simulink library "microgridLib"  (R2023a)
settings: Solver=VariableStepAuto  StartTime=0.0  StopTime=10.0  RelTol=1e-3
values from neighbouring files (symbols this model uses):
  Ts = 5.0E-5    [microgrid_system.sldd]
  Ts_Control = 5.0E-5    [microgrid_system.sldd]
undefined symbols (not defined in the file or in its folder): BR, D1, Delta, DiscIntNeverNeededParam, fnom, gcbh, I1_init, Ion, j, Lithium, Mag_V0, np, nq, Pha_V0, PQext, sps_rtmsupport, Tp1, Tp2, Tq1, Tq2, Vbase, Vmin, Vnom
libraries: slpidlib x11, spsThreePhaseSeriesRLCBranchLib x10, spsGroundLib x9, spsVoltageMeasurementLib x7, spsSeriesRLCBranchLib x7, spsControlledCurrentSourceLib x6, spsabctodq0Lib x6, spsFourierLib x5, spsPower3phInstantaneousLib x5, spsThreePhaseSeriesRLCLoadLib x4, spsThreePhaseTransformerTwoWindingsLib x4, spsThreePhaseVIMeasurementLib x3
(part 1 of 4)
settings Model: Creator=Jon  LastModifiedBy=steve.liu
settings SolverCC: AlgebraicLoopSolver=TrustRegion
settings DataIOCC: ReturnWorkspaceOutputs=off
settings DebuggingCC: UnconnectedInputMsg=warning  UnconnectedOutputMsg=warning  UnconnectedLineMsg=warning  ArithmeticOperatorsInVariantConditions=warning
settings ModelReferenceCC: EnableRefExpFcnMdlSchedulingChecks=on
settings SFSimCC: SimUseLocalCustomCode=off  CustomCodeUndefinedFunction=UseInterfaceOnly
settings RTWCC: RTWUseLocalCustomCode=off  DLArmComputeVersion=19.05
settings CodeAppCC: StateflowObjectComments=on

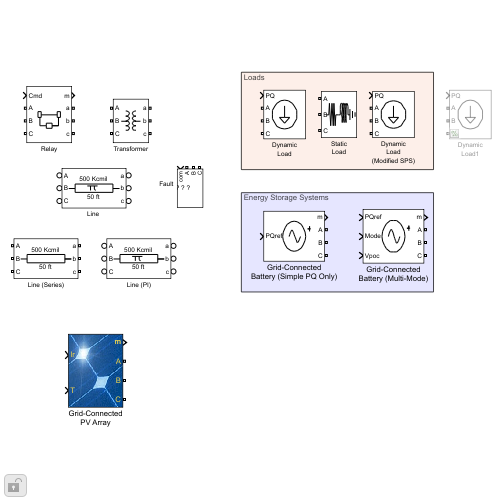
[thumbnail: Simulink's stored preview of the top-level diagram]
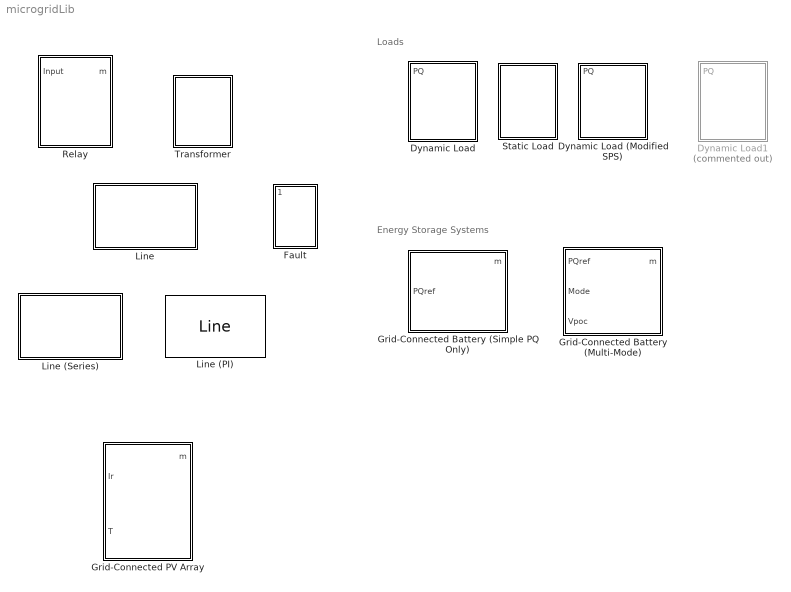
== system microgridLib ==
  note: Energy Storage Systems
  note: Loads
  Dynamic Load : Subsystem  mask{Vrms=460, Freq=60, Ts=Ts, Tau=1e-4}
      mask prompts: Vrms "Nominal L-L Voltage, Vrms"; Freq "Nominal Frequency, Hz"; Ts "Sample Rate, s"; Tau "Algebraic Loop Time Constant, Tau [s]"
      mask Display:
      | plot(-45,-45,45,45,[0,9,18,24,29,30,29,24,18,9,0,-9,-18,-24,-29,-30,-29,-24,-18,-9,0]*.9,[30,29,24,18,9,0,-9,-18,-24,-29,-30,-29,-24,-18,-9,0,9,18,24,29,30]*.9)
      | plot([0,0,10,0,-10,0]*1.1,[15,-5,-5,-15,-5,-5]*1.1)
      | 
      | port_label('input', 1, 'PQ')
      | port_label('LConn', 1, 'A')
      | port_label('LConn', 2, 'B')
      | port_label('LConn', 3, 'C')
  Dynamic Load (Modified SPS) : Subsystem  mask{Vrms=460, Freq=60, PQ0=[100 10]}
      mask prompts: Vrms "Nominal L-L Voltage, Vrms"; Freq "Nominal Frequency"; PQ0 "[P0 Q0]"
      mask init:
      | P0 = PQ0(1);
      | Q0 = PQ0(2);
      mask Display:
      | plot(-45,-45,45,45,[0,9,18,24,29,30,29,24,18,9,0,-9,-18,-24,-29,-30,-29,-24,-18,-9,0]*.9,[30,29,24,18,9,0,-9,-18,-24,-29,-30,-29,-24,-18,-9,0,9,18,24,29,30]*.9)
      | plot([0,0,10,0,-10,0]*1.1,[15,-5,-5,-15,-5,-5]*1.1)
      | 
      | port_label('input', 1, 'PQ')
      | port_label('LConn', 1, 'A')
      | port_label('LConn', 2, 'B')
      | port_label('LConn', 3, 'C')
  Dynamic Load1 : Subsystem  Commented=on  mask{Vrms=460, Freq=60, Ts=Ts, Tau=1e-4}
      mask prompts: Vrms "Nominal L-L Voltage, Vrms"; Freq "Nominal Frequency, Hz"; Ts "Sample Rate, s"; Tau "Algebraic Loop Time Constant, Tau [s]"
      mask Display:
      | plot(-45,-45,45,45,[0,9,18,24,29,30,29,24,18,9,0,-9,-18,-24,-29,-30,-29,-24,-18,-9,0]*.9,[30,29,24,18,9,0,-9,-18,-24,-29,-30,-29,-24,-18,-9,0,9,18,24,29,30]*.9)
      | plot([0,0,10,0,-10,0]*1.1,[15,-5,-5,-15,-5,-5]*1.1)
      | 
      | port_label('input', 1, 'PQ')
      | port_label('LConn', 1, 'A')
      | port_label('LConn', 2, 'B')
      | port_label('LConn', 3, 'C')
  "Fault " : Subsystem  DialogController=POWERSYS.PowerSysDialog  LoadFcn=sps_rtmsupport('LoadFcn',gcbh);  StartFcn=sps_rtmsupport('StartFcn',gcbh);  StopFcn=sps_rtmsupport('StopFcn',gcbh);  mask(Three-Phase Fault){InitialStates=0, FaultA=on, FaultB=on, FaultC=on, GroundFault=on, SwitchTimes=[ 1/60 6/60], External=on, SwitchStatus=NaN, FaultResistance=0.01, GroundResistance=0.001, SnubberResistance=inf, SnubberCapacitance=inf, Measurements=Fault currents}
      mask prompts: InitialStates "Initial status:"; FaultA "Phase A"; FaultB "Phase B"; FaultC "Phase C"; GroundFault "Ground"; SwitchTimes "Switching times (s):"; SwitchStatus "Transition status:"; FaultResistance "Fault resistance Ron (Ohm):"; GroundResistance "Ground resistance Rg (Ohm):"; SnubberResistance "Snubber resistance Rs (Ohm):"; SnubberCapacitance "Snubber capacitance Cs (F):"
      mask help: Implements a fault (short-circuit) between any phase and the ground. When the external switching time mode is selected, a Simulink logical signal is used to control the fault operation.
      mask init:
      | block = gcb;
      | [FaultIcon,FaultA,FaultB,FaultC,GroundResistance,initialA,initialB,initialC,Ts,SwitchTimes,SwitchStatus] = powericon('ThreePhaseFaultInit',block,GroundResistance,SwitchTimes,SwitchStatus,FaultA,FaultB,FaultC,GroundFault,InitialStates,External);
      | powericon('ThreePhaseFaultCback',block);
      settings: CopyFcn=sps_rtmsupport('CopyFcn',gcbh);  DeleteFcn=sps_rtmsupport('DeleteFcn',gcbh);  UndoDeleteFcn=sps_rtmsupport('UndoDeleteFcn',gcbh);  ModelCloseFcn=sps_rtmsupport('ModelCloseFcn',gcbh);  PreSaveFcn=sps_rtmsupport('PreSaveFcn',gcbh);  PostSaveFcn=sps_rtmsupport('PostSaveFcn',gcbh);  NameChangeFcn=sps_rtmsupport('NameChangeFcn',gcbh);  PreCopyFcn=sps_rtmsupport('PreCopyFcn',gcbh);  OpenFcn=sps_rtmsupport('OpenFcn',gcbh, [ 2 3 4 5 7 13]);  CloseFcn=sps_rtmsupport('CloseFcn',gcbh);  PreDeleteFcn=sps_rtmsupport('PreDeleteFcn',gcbh);
      mask Help: helpview(psbhelp)
      mask Callback GroundFault: powericon('ThreePhaseFaultCback',gcb);
      mask Callback External: powericon('ThreePhaseFaultCback',gcb);
      mask TypeOptions Measurements: None | Fault voltages | Fault currents | Fault voltages and currents
      mask DialogControl Container3 Prompt: Fault between:
      mask Display:
      | image(imread(FaultIcon,'bmp'))
      | port_label('LConn', 1, 'A')
      | port_label('LConn', 2, 'B')
      | port_label('LConn', 3, 'C')
  Grid-Connected Battery (Multi-Mode) : Subsystem  mask{Pmod=25, Vnom_dc=480, Bcap=500, Vnom_prim=4600, Fnom=60, Ts=Ts, Ts_Control=Ts_Control}
      mask prompts: Pmod "Scale Battery, Multiplier for 100 kW"; Vnom_dc "Nominal Battery Voltage, V"; Bcap "Battery Capacity, Ah"; Vnom_prim "Nominal Grid Connection L-L Voltage, Vrms"; Fnom "Grid Frequency, Fnom [Hz]"; Ts "Simulation Time Step, Ts [s]"; Ts_Control "Controller Time Step, Ts_Control"
      mask init:
      | Pnom = Pmod*100e3;      % Inverter nominal 3-phase power (VA)
      | Vnom_dc = 480;     % Nominal DC link voltage (V)
      | % Vnom_prim = 25e3;  % Nominal inverter primary line-to-line voltage(Vrms)
      | Vnom_sec= 0.85*Vnom_dc/2/sqrt(2)*sqrt(3); % Nominal inverter secondary line-to-line voltage (Vrms)
      | 
      | TotalLeakage = 0.06;   % Transformer total leakage (pu)
      | Rxf = TotalLeakage/25;
      | Lxf = TotalLeakage;
      | 
      | % Inverter choke RL [Rpu Lpu]
      | Rchoke = 0.15/100;
      | Lchoke = 0.15;
      | Zbase = Vnom_sec^2/Pnom;
      | 
      | % Filter C Parameters
      | Qc = 0.1*Pnom;     % Capacitive reactive power (var)
      | Pc = Qc/50;        % Active power (W)      
      | 
      | Clink = 2 * 3/4 * (Pnom/Fnom*2/Vnom_dc^2); % DC link energy for 3/4 cycle of Pnom
      | 
      | % VDC regulator (VDCreg)
      | Kp_VDCreg = 2;           % Proportional gain
      | Ki_VDCreg = 400;        % Integral gain
      | 
      | Rtot_pu = Rxf + Rchoke; % Feedforward values
      | Ltot_pu = Lxf + Lchoke; % Feedforward values
      | 
      | Kp_Ireg = 0.3;          % Proportional gain
      | Ki_Ireg = 20;           % Integral gain
      settings: LibrarySourceBlock=|
      | microgridLib/Grid-Connected
      | Battery (Multi-Mode)
      mask Display: plot(-80,-50,80,50,[0,9,18,24,29,30,29,24,18,9,0,-9,-18,-24,-29,-30,-29,-24,-18,-9,0],[30,29,24,18,9,0,-9,-18,-24,-29,-30,-29,-24,-18,-9,0,9,18,24,29,30],[-50],[0],[50],[0],[45 35 40 40 40],[15 15 15 20 10],[1 2 3 4 5 6 7 8 9 10 11 12 13 14 15 16 17 18 19 20 21].*1.5-15,[0,9,18,24,29,30,29,24,18,9,0,-9,-18,-24,-29,-30,-29,-24,-18,-9,0]./2.4)
  Grid-Connected Battery (Simple PQ Only) : Subsystem  mask{Pmod=15, Vnom_dc=480, Bcap=500, Vnom_prim=2400, Fnom=60, Ts=Ts, Ts_Control=Ts_Control}
      mask prompts: Pmod "Scale Battery, Multiplier for 100 kW"; Vnom_dc "Nominal Battery Voltage, V"; Bcap "Battery Capacity, Ah"; Vnom_prim "Nominal Grid Connection L-L Voltage, Vrms"; Fnom "Grid Frequency, Fnom [Hz]"; Ts "Simulation Time Step, Ts [s]"; Ts_Control "Controller Time Step, Ts_Control"
      mask init: same as microgridLib/Grid-Connected Battery (Multi-Mode)
      mask Display: plot(-80,-50,80,50,[0,9,18,24,29,30,29,24,18,9,0,-9,-18,-24,-29,-30,-29,-24,-18,-9,0],[30,29,24,18,9,0,-9,-18,-24,-29,-30,-29,-24,-18,-9,0,9,18,24,29,30],[-50],[0],[50],[0],[45 35 40 40 40],[15 15 15 20 10],[1 2 3 4 5 6 7 8 9 10 11 12 13 14 15 16 17 18 19 20 21].*1.5-15,[0,9,18,24,29,30,29,24,18,9,0,-9,-18,-24,-29,-30,-29,-24,-18,-9,0]./2.4)
  Grid-Connected PV Array : Subsystem  mask{Pmod=5, Vnom_prim=2400, Fnom=60, Ts=Ts, Ts_Control=Ts_Control}
      mask prompts: Pmod "Scale Array, Multiplier for 100 kW"; Vnom_prim "Nominal Grid Connection L-L Voltage, Vrms"; Fnom "Grid Frequency, Fnom [Hz]"; Ts "Simulation Time Step, Ts [s]"; Ts_Control "Controller Time Step, Ts_Control"
      mask init:
      | Pnom = Pmod*100e3;      % Inverter nominal 3-phase power (VA)
      | Vnom_dc = 480;     % Nominal DC link voltage (V)
      | % Vnom_prim = 25e3;  % Nominal inverter primary line-to-line voltage(Vrms)
      | Vnom_sec= 0.85*Vnom_dc/2/sqrt(2)*sqrt(3); % Nominal inverter secondary line-to-line voltage (Vrms)
      | 
      | TotalLeakage = 0.06;   % Transformer total leakage (pu)
      | Rxf = TotalLeakage/25;
      | Lxf = TotalLeakage;
      | 
      | % Inverter choke RL [Rpu Lpu]
      | Rchoke = 0.15/100;
      | Lchoke = 0.15;
      | Zbase = Vnom_sec^2/Pnom;
      | 
      | % Filter C Parameters
      | Qc = 0.1*Pnom;     % Capacitive reactive power (var)
      | Pc = Qc/50;        % Active power (W)      
      | 
      | Clink = 2 * 3/4 * (Pnom/Fnom*2/Vnom_dc^2); % DC link energy for 3/4 cycle of Pnom
      | 
      | % MPPT Control (Perturb & Observe Algorithm)
      | Increment_MPPT = 0.01;     % Increment value used to increase/decrease Vdc_ref
      | Limits_MPPT = [ 1.25*Vnom_dc 0.75*Vnom_dc ]; % Upper & Lower limit for Vdc_ref (V)
      | 
      | % VDC regulator (VDCreg)
      | Kp_VDCreg = 2;           % Proportional gain
      | Ki_VDCreg = 400;        % Integral gain
      | 
      | Rtot_pu = Rxf + Rchoke; % Feedforward values
      | Ltot_pu = Lxf + Lchoke; % Feedforward values
      | 
      | Kp_Ireg = 0.3;          % Proportional gain
      | Ki_Ireg = 20;           % Integral gain
      settings: LibrarySourceBlock=|
      | microgridLib/Grid-Connected
      | PV Array
      mask Display:
      | image('panel.jpg')
      | color('yellow')
      | port_label('input',1,'Ir')
      | port_label('input',2,'T')
      | port_label('output',1,'m')
      | port_label('output',1,'m')
      | port_label('Rconn',1,'A')
      | port_label('Rconn',2,'B')
      | port_label('Rconn',3,'C')
  "Line " : Subsystem  mask{gauge=500 Kcmil, Freq=60, Length_ft=50, Ratio=3}
      mask prompts: gauge "Line Gauge"; Freq "Nominal Frequency, Hz"; Length_ft "Length, ft"; Ratio "Ratio Impedance, Z0/Z1"
      mask init:
      | Length = 0.0003048*Length_ft; % ft/km
      | 
      | MaskVals = get_param(gcb,'MaskValues');
      | GaugeStr = MaskVals{1};
      | LengthStr = MaskVals{3};
      | 
      | switch gauge
      |     case 1  %500 Kcmil
      |         R0 = 0.0965;        L0 = 3.0372e-04;        
      |     case 2  %350 Kcmil
      |         R0 = 0.1240;        L0 = 3.2461e-04; 
      |     case 3  %4/0 AWG
      |         R0 = 0.2100;        L0 = 3.3156e-04; 
      |     case 4  %3/0 AWG
      |         R0 = 0.2653;        L0 = 3.3800e-04;
      |     case 5  %2/0 AWG
      |         R0 = 0.3346;        L0 = 3.5420e-04; 
      |     case 6  %1/0 AWG
      |         R0 = 0.4199;        L0 = 3.6030e-04;
      | end
      | 
      | % Zero-sequence Parameters
      | R1 = R0/Ratio;
      | L1 = L0/Ratio;
      mask TypeOptions gauge: 500 Kcmil | 350 Kcmil | 4/0 AWG | 3/0 AWG | 2/0 AWG | 1/0 AWG
      mask Display:
      | plot(0,0,1,1,[.20,.20,.80,.80,.90,.80,.80,.20,.20,.10],[.50,.40,.40,.50,.50,.50,.61,.61,.50,.50],[.56,.39],[.55,.55],[.44,.44],[.44,.55],[.53,.50,.50],[.44,.48,.55])
      | 
      | text(0.5,0.75,GaugeStr,'horizontalAlignment', 'center');
      | text(0.5,0.3,[LengthStr ' ft'],'horizontalAlignment', 'center');
      | 
      | 
      | port_label('RConn', 1, 'a')
      | port_label('RConn', 2, 'b')
      | port_label('RConn', 3, 'c')
      | port_label('LConn', 1, 'A')
      | port_label('LConn', 2, 'B')
      | port_label('LConn', 3, 'C')
  Line (PI) : $bdroot/Line   gauge=500 Kcmil  Freq=60  Length_ft=50  Ratio=3
  Line (Series) : Subsystem  mask{gauge=500 Kcmil, Length=50}
      mask prompts: gauge "Line Gauge"; Length "Length, ft"
      mask init:
      | MaskVals = get_param(gcb,'MaskValues');
      | GaugeStr = MaskVals{1};
      | LengthStr = MaskVals{2};
      | 
      | switch gauge
      |     case 1  %500 Kcmil
      |         R0 = 2.94e-5;       L0 = 9.2575e-8;        
      |     case 2  %350 Kcmil
      |         R0 = 3.78e-5;       L0 = 9.8941e-8; 
      |     case 3  %4/0 AWG
      |         R0 = 6.4e-5;        L0 = 1.03-07; 
      |     case 4  %3/0 AWG
      |         R0 = 7.61e-5;       L0 = 1.05e-7;
      |     case 5  %2/0 AWG
      |         R0 = 1.02e-4;       L0 = 1.0796e-7; 
      |     case 6  %1/0 AWG
      |         R0 = 1.28e-4;       L0 = 1.0982e-7;
      | end
      | 
      | R0 = R0;
      | L0 = L0;
      mask TypeOptions gauge: 500 Kcmil | 350 Kcmil | 4/0 AWG | 3/0 AWG | 2/0 AWG | 1/0 AWG
      mask Display:
      | plot(0,0,1,1,[.20,.20,.80,.80,.90,.80,.80,.20,.20,.10],[.50,.40,.40,.50,.50,.50,.61,.61,.50,.50])
      | 
      | text(0.5,0.75,GaugeStr,'horizontalAlignment', 'center');
      | text(0.5,0.3,[LengthStr ' ft'],'horizontalAlignment', 'center');
      | 
      | 
      | port_label('RConn', 1, 'a')
      | port_label('RConn', 2, 'b')
      | port_label('RConn', 3, 'c')
      | port_label('LConn', 1, 'A')
      | port_label('LConn', 2, 'B')
      | port_label('LConn', 3, 'C')
  Relay : Subsystem
      mask Display:
      | X.p1 = -20;
      | X.p2 = 120;
      | Y.p1 = 0;
      | Y.p2 = 100;
      | X.p3 = [15,15,25,25,15];
      | Y.p3 = [55,45,45,55,55];
      | X.p4 = [75,75,85,85,75];
      | Y.p4 = [55,45,45,55,55];
      | X.p5 = [25,75];
      | Y.p5 = [50,50];
      | X.p6 = [20,20,40,40,60,60,80,80,80,60,60,40,40];
      | Y.p6 = [45,30,30,35,35,30,30,45,30,30,25,25,30];
      | plot(X.p1,Y.p1,X.p2,Y.p2,X.p3,Y.p3,X.p4,Y.p4,X.p5,Y.p5,X.p6,Y.p6)
      | 
      | port_label('input',1','Cmd');
      | port_label('output',1,'m');
      | 
      | port_label('RConn', 1, 'a')
      | port_label('RConn', 2, 'b')
      | port_label('RConn', 3, 'c')
      | port_label('LConn', 1, 'A')
      | port_label('LConn', 2, 'B')
      | port_label('LConn', 3, 'C')
  Static Load : Subsystem  mask{kS=100, PF=0.9, Vrms=460, Freq=60}
      mask prompts: kS "Complex Power, kVA"; PF "Power Factor, PF"; Vrms "Nominal L-L Voltage, Vrms"; Freq "Nominal Frequency"
      mask init:
      | S = 1000*kS;
      mask Display:
      | rx  = [0 30 30 38 53 68 83 98 113 120 120 150];
      | ry  = [0 0 0 25 -25 25 -25 25 -25 0 0 0];
      | 
      | lx  = [0 23 23 24 28 34 40 47 52 55 56 54 51 51 47 46 48 51 57 64 70 75 79 79 77 74 74 70 69 71 75 80 87 93 99 102 103 101 97 97 94 93 94 98 104 110 117 122 125 126 126 150];
      | ly  = [0 0 1 11 19 24 25 23 17 8 -2 -12 -18 -18 -9 1 11 19 24 25 23 17 8 -2 -12 -18 -18 -9 1 11 19 24 25 23 17 8 -2 -12 -18 -18 -9 1 11 19 24 25 23 17 8 0 0 0];
      | 
      | s1 = 0;
      | s2 = -50;
      | s3 = 300;
      | s4 = 50;
      | r1 = rx;
      | r2 = ry;
      | l1 = lx+150;
      | l2 = ly;
      | 
      | plot(s1-60,s2,s3+80,s4,r1,r2,l1,l2)
      | 
      | plot( [s3,s3], [-s2/4,s2/4])
      | plot( [s3+30,s3+30], [-s2/6,s2/6])
      | plot( [s3+60,s3+60], [-s2/10,s2/10])
      | 
      | port_label('LConn', 1, 'A')
      | port_label('LConn', 2, 'B')
      | port_label('LConn', 3, 'C')
  Transformer : Subsystem  mask{kS=225, Freq=60, Vp=4160, Vs=460, Zperc=5.18, Ratio=2.5}
      mask prompts: kS "Nominal Power, kVA"; Freq "Nominal Frequency, Hz"; Vp "Primary L-L Voltage, Vrms"; Vs "Secondary L-L Voltage, Vrms"; Zperc "Impedance - Z, %"; Ratio "X/R Ratio"
      mask init:
      | S = kS*1000;
      | Z = Zperc/100;
      mask Display:
      | plot(-180,-220,180,220,[-100,-40],[0,0],[100,40],[0,0],[2 42 74 94 100 90 66 30 0 2 42 74 94 100 90 66 30 0 2 42 74 94 100 90 66 30 0 2 42 74 94 100 90 66 30 0]*.4-55,[-45 -45 -34 -17 3 22 38 48 50 50 55 66 83 103 122 138 148 150 150 155 166 183 203 222 238 248 250 250 255 266 283 303 322 338 348 348]*0.5-75,[2 42 74 94 100 90 66 30 0 2 42 74 94 100 90 66 30 0 2 42 74 94 100 90 66 30 0 2 42 74 94 100 90 66 30 0]*-.4+55,[-45 -45 -34 -17 3 22 38 48 50 50 55 66 83 103 122 138 148 150 150 155 166 183 203 222 238 248 250 250 255 266 283 303 322 338 348 348]*0.5-75)
      | 
      | 
      | port_label('RConn', 1, 'a')
      | port_label('RConn', 2, 'b')
      | port_label('RConn', 3, 'c')
      | port_label('LConn', 1, 'A')
      | port_label('LConn', 2, 'B')
      | port_label('LConn', 3, 'C')

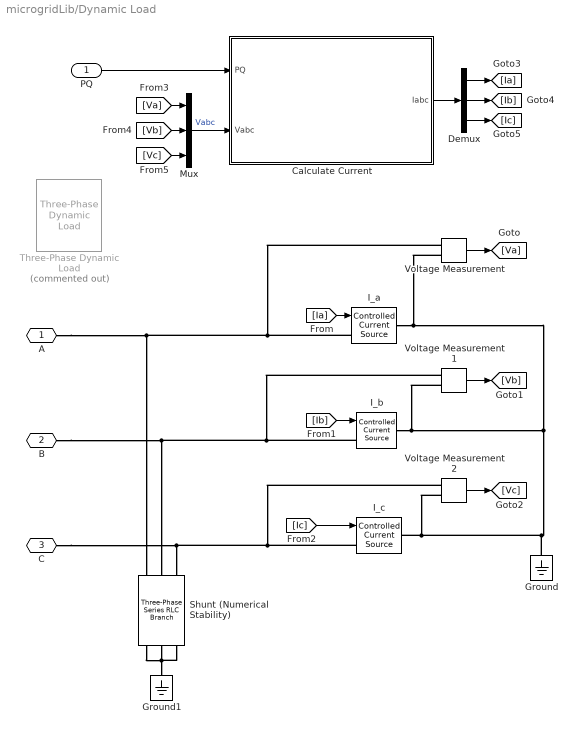
== system microgridLib/Dynamic Load ==
  PQ : Inport
  Calculate Current : Subsystem
  Demux : Demux  Outputs=3
  Ground : spsGroundLib/Ground  LConnTagsString=a
  Ground1 : spsGroundLib/Ground  LConnTagsString=a
  I_a : spsControlledCurrentSourceLib/Controlled Current Source  Initialize=off  Source_Type=AC  Amplitude=0  Phase=0  Frequency=0  Measurements=None
  I_b : spsControlledCurrentSourceLib/Controlled Current Source  Initialize=off  Source_Type=AC  Amplitude=0  Phase=0  Frequency=0  Measurements=None
  I_c : spsControlledCurrentSourceLib/Controlled Current Source  Initialize=off  Source_Type=AC  Amplitude=0  Phase=0  Frequency=0  Measurements=None
  Mux : Mux  Inputs=3
  Shunt (Numerical Stability) : spsThreePhaseSeriesRLCBranchLib/Three-Phase Series RLC Branch  LConnTagsString=A|B|C  RConnTagsString=A|B|C  BranchType=R  Resistance=1e7  Inductance=1e-3  Capacitance=1e-6  Measurements=None
  Three-Phase Dynamic Load : spsThreePhaseDynamicLoadLib/Three-Phase Dynamic Load  Commented=on  NominalVoltage=[ Vrms Freq ]  ActiveReactivePowers=[0 0]  PositiveSequence=[0.994 -11.8]  ExternalControl=on  NpNq=[1.3 2]  TimeConstants="[0  0  0  0]"  MinimumVoltage=0.7  Tfilter=Tau  LoadFlowParameters=[4,0,0,0,0]
      settings: LibrarySourceBlock=|
      | sps_lib/Passives/Three-Phase
      | Dynamic Load
  Voltage Measurement : spsVoltageMeasurementLib/Voltage Measurement  PhasorSimulation=off  OutputType=Complex  PSBequivalent=0
  Voltage Measurement1 : spsVoltageMeasurementLib/Voltage Measurement  PhasorSimulation=off  OutputType=Complex  PSBequivalent=0
  Voltage Measurement2 : spsVoltageMeasurementLib/Voltage Measurement  PhasorSimulation=off  OutputType=Complex  PSBequivalent=0
  A : PMIOPort  Side=Left
  B : PMIOPort  Port=2  Side=Left
  C : PMIOPort  Port=3  Side=Left
  wires:
  Voltage Measurement/1 -> [Va]
  Demux/2 -> [Ib]
  Mux/1 -> Calculate Current/2(Vabc)  "Vabc"
  Voltage Measurement1/1 -> [Vb]
  [Va] -> Mux/1
  Demux/1 -> [Ia]
  Calculate Current/1(Iabc) -> Demux/1
  [Ia] -> I_a/1
  Voltage Measurement2/1 -> [Vc]
  [Vb] -> Mux/2
  [Vc] -> Mux/3
  Demux/3 -> [Ic]
  [Ib] -> I_b/1
  [Ic] -> I_c/1
  PQ/1 -> Calculate Current/1(PQ)
  connections:
  Shunt (Numerical Stability)/RConn3 -- Shunt (Numerical Stability)/RConn1 -- Shunt (Numerical Stability)/RConn2 -- Ground1/LConn1
  Voltage Measurement/LConn1 -- I_a/LConn1 -- Shunt (Numerical Stability)/LConn1 -- A/RConn1
  I_b/LConn1 -- Voltage Measurement1/LConn1 -- B/RConn1 -- Shunt (Numerical Stability)/LConn2
  Voltage Measurement2/LConn1 -- I_c/LConn1 -- C/RConn1 -- Shunt (Numerical Stability)/LConn3
  Ground/LConn1 -- Voltage Measurement/LConn2 -- I_a/RConn1 -- I_b/RConn1 -- Voltage Measurement1/LConn2 -- I_c/RConn1 -- Voltage Measurement2/LConn2

== system microgridLib/Dynamic Load (Modified SPS) ==
  PQ : Inport
  Ground : spsGroundLib/Ground  LConnTagsString=a
  Shunt (Numerical Stability) : spsThreePhaseSeriesRLCBranchLib/Three-Phase Series RLC Branch  LConnTagsString=A|B|C  RConnTagsString=A|B|C  BranchType=R  Resistance=1e9  Inductance=1e-3  Capacitance=1e-6  Measurements=None
  Terminator : Terminator
  Three-Phase Dynamic Load : Subsystem  Commented=on  DialogController=POWERSYS.PowerSysDialog  LoadFcn=sps_rtmsupport('LoadFcn',gcbh);  StartFcn=sps_rtmsupport('StartFcn',gcbh);  StopFcn=sps_rtmsupport('StopFcn',gcbh);  mask(Three-Phase Dynamic Load){NominalVoltage=[Vrms Freq], ActiveReactivePowers=[P0 Q0], PositiveSequence=[0.994 -11.8], ExternalControl=on, NpNq=[1.3 2], TimeConstants=[0  0  0  0], MinimumVoltage=0.7, Tfilter=1e-4, LoadFlowParameters=[4,0,0,0,0]}
      mask prompts: NominalVoltage "Nominal L-L voltage and frequency  [Vn(Vrms) fn(Hz)]:"; ActiveReactivePowers "Active and reactive power at initial voltage [Po(W) Qo(var)]:"; PositiveSequence "Initial positive-sequence voltage Vo [Mag(pu) Phase (deg.)]:"; ExternalControl "External control of PQ"; NpNq "[np, nq]:"; TimeConstants "Time constants [Tp1 Tp2 Tq1 Tq2]  (s):"; MinimumVoltage "Minimum voltage Vmin (pu):"; Tfilter "Filtering time constant (s):"; LoadFlowParameters "Load Flow parameters"
      mask help: Implements a three-phase, three-wire dynamic load. Active power P and reactive power Q absorbed by the load vary as function of positive-sequence voltage V.
      mask init:
      | block = gcb;
      | [Ts, WantBlockChoice, Vnom,fnom,P0,Q0,Mag_V0,Pha_V0,V0_d,V0_q,np,nq,Tp1,Tp2,Tq1,Tq2,Vbase,I1_init,Mag_ia,Phase_ia,Vmin,PQext,a] = powericon('ThreePhaseDynamicLoadInit',block,NominalVoltage,ActiveReactivePowers,PositiveSequence,NpNq,TimeConstants,MinimumVoltage,ExternalControl);
      | powericon('SetInternalModels','set',block,WantBlockChoice);
      settings: CopyFcn=sps_rtmsupport('CopyFcn',gcbh); powericon('psbloadfunction',gcb,'gotofrom','UpdateGotoTag');  DeleteFcn=sps_rtmsupport('DeleteFcn',gcbh);  UndoDeleteFcn=sps_rtmsupport('UndoDeleteFcn',gcbh);  ModelCloseFcn=sps_rtmsupport('ModelCloseFcn',gcbh);  PreSaveFcn=sps_rtmsupport('PreSaveFcn',gcbh);  PostSaveFcn=sps_rtmsupport('PostSaveFcn',gcbh);  NameChangeFcn=sps_rtmsupport('NameChangeFcn',gcbh);  PreCopyFcn=sps_rtmsupport('PreCopyFcn',gcbh);  OpenFcn=sps_rtmsupport('OpenFcn',gcbh, 4);  CloseFcn=sps_rtmsupport('CloseFcn',gcbh);  PreDeleteFcn=sps_rtmsupport('PreDeleteFcn',gcbh);
      mask Help: helpview(psbhelp)
      mask Callback ExternalControl: %powericon('ThreePhaseDynamicLoadCback',gcb);
      mask Display:
      | plot(-45,-45,45,45,[0,9,18,24,29,30,29,24,18,9,0,-9,-18,-24,-29,-30,-29,-24,-18,-9,0]*.9,[30,29,24,18,9,0,-9,-18,-24,-29,-30,-29,-24,-18,-9,0,9,18,24,29,30]*.9)
      | plot([0,0,10,0,-10,0]*1.1,[15,-5,-5,-15,-5,-5]*1.1)
  Three-Phase Dynamic Load (custom) : Subsystem  DialogController=POWERSYS.PowerSysDialog  LoadFcn=sps_rtmsupport('LoadFcn',gcbh);  StartFcn=sps_rtmsupport('StartFcn',gcbh);  StopFcn=sps_rtmsupport('StopFcn',gcbh);  mask(Three-Phase Dynamic Load){NominalVoltage=[ 460 60 ], ActiveReactivePowers=[P0 Q0], PositiveSequence=[0.994 -11.8], ExternalControl=on, NpNq=[1.3 2], TimeConstants=[0  0  0  0], MinimumVoltage=0.7, Tfilter=1e-4, LoadFlowParameters=[4,0,0,0,0]}
      mask prompts: NominalVoltage "Nominal L-L voltage and frequency  [Vn(Vrms) fn(Hz)]:"; ActiveReactivePowers "Active and reactive power at initial voltage [Po(W) Qo(var)]:"; PositiveSequence "Initial positive-sequence voltage Vo [Mag(pu) Phase (deg.)]:"; ExternalControl "External control of PQ"; NpNq "[np, nq]:"; TimeConstants "Time constants [Tp1 Tp2 Tq1 Tq2]  (s):"; MinimumVoltage "Minimum voltage Vmin (pu):"; Tfilter "Filtering time constant (s):"; LoadFlowParameters "Load Flow parameters"
      mask help: Implements a three-phase, three-wire dynamic load. Active power P and reactive power Q absorbed by the load vary as function of positive-sequence voltage V.
      mask init:
      | block = gcb;
      | [Ts, WantBlockChoice, Vnom,fnom,P0,Q0,Mag_V0,Pha_V0,V0_d,V0_q,np,nq,Tp1,Tp2,Tq1,Tq2,Vbase,I1_init,Mag_ia,Phase_ia,Vmin,PQext,a] = powericon('ThreePhaseDynamicLoadInit',block,NominalVoltage,ActiveReactivePowers,PositiveSequence,NpNq,TimeConstants,MinimumVoltage,ExternalControl);
      | %powericon('SetInternalModels','set',block,WantBlockChoice);
      settings: CopyFcn=sps_rtmsupport('CopyFcn',gcbh); powericon('psbloadfunction',gcb,'gotofrom','UpdateGotoTag');  DeleteFcn=sps_rtmsupport('DeleteFcn',gcbh);  UndoDeleteFcn=sps_rtmsupport('UndoDeleteFcn',gcbh);  ModelCloseFcn=sps_rtmsupport('ModelCloseFcn',gcbh);  PreSaveFcn=sps_rtmsupport('PreSaveFcn',gcbh);  PostSaveFcn=sps_rtmsupport('PostSaveFcn',gcbh);  NameChangeFcn=sps_rtmsupport('NameChangeFcn',gcbh);  PreCopyFcn=sps_rtmsupport('PreCopyFcn',gcbh);  OpenFcn=sps_rtmsupport('OpenFcn',gcbh, 4);  CloseFcn=sps_rtmsupport('CloseFcn',gcbh);  PreDeleteFcn=sps_rtmsupport('PreDeleteFcn',gcbh);
      mask Help: helpview(psbhelp)
      mask Callback ExternalControl: %powericon('ThreePhaseDynamicLoadCback',gcb);
      mask Display:
      | plot(-45,-45,45,45,[0,9,18,24,29,30,29,24,18,9,0,-9,-18,-24,-29,-30,-29,-24,-18,-9,0]*.9,[30,29,24,18,9,0,-9,-18,-24,-29,-30,-29,-24,-18,-9,0,9,18,24,29,30]*.9)
      | plot([0,0,10,0,-10,0]*1.1,[15,-5,-5,-15,-5,-5]*1.1)
  kW_kVAr_per_phase1 : Gain  Commented=on  Gain=1000
  A : PMIOPort  Side=Left
  B : PMIOPort  Port=2  Side=Left
  C : PMIOPort  Port=3  Side=Left
  wires:
  Three-Phase Dynamic Load (custom)/1(m) -> Terminator/1
  PQ/1 -> Three-Phase Dynamic Load (custom)/1(PQ)
  connections:
  B/RConn1 -- Three-Phase Dynamic Load (custom)/LConn2 -- Shunt (Numerical Stability)/LConn2
  A/RConn1 -- Three-Phase Dynamic Load (custom)/LConn1 -- Shunt (Numerical Stability)/LConn1
  C/RConn1 -- Three-Phase Dynamic Load (custom)/LConn3 -- Shunt (Numerical Stability)/LConn3
  Ground/LConn1 -- Shunt (Numerical Stability)/RConn3 -- Shunt (Numerical Stability)/RConn2 -- Shunt (Numerical Stability)/RConn1

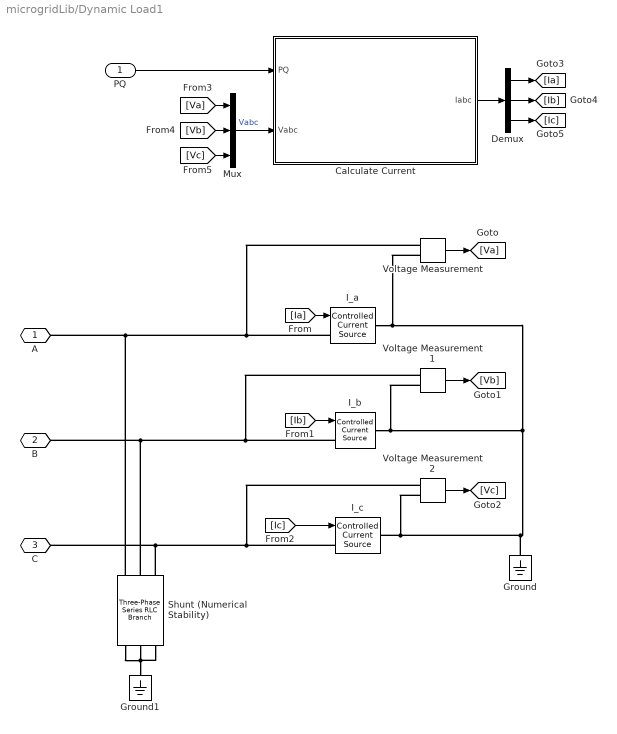
== system microgridLib/Dynamic Load1 ==
  PQ : Inport
  Calculate Current : Subsystem
  Demux : Demux  Outputs=3
  Ground : spsGroundLib/Ground  LConnTagsString=a
  Ground1 : spsGroundLib/Ground  LConnTagsString=a
  I_a : spsControlledCurrentSourceLib/Controlled Current Source  Initialize=off  Source_Type=AC  Amplitude=0  Phase=0  Frequency=0  Measurements=None
  I_b : spsControlledCurrentSourceLib/Controlled Current Source  Initialize=off  Source_Type=AC  Amplitude=0  Phase=0  Frequency=0  Measurements=None
  I_c : spsControlledCurrentSourceLib/Controlled Current Source  Initialize=off  Source_Type=AC  Amplitude=0  Phase=0  Frequency=0  Measurements=None
  Mux : Mux  Inputs=3
  Shunt (Numerical Stability) : spsThreePhaseSeriesRLCBranchLib/Three-Phase Series RLC Branch  LConnTagsString=A|B|C  RConnTagsString=A|B|C  BranchType=R  Resistance=1e7  Inductance=1e-3  Capacitance=1e-6  Measurements=None
  Voltage Measurement : spsVoltageMeasurementLib/Voltage Measurement  PhasorSimulation=off  OutputType=Complex  PSBequivalent=0
  Voltage Measurement1 : spsVoltageMeasurementLib/Voltage Measurement  PhasorSimulation=off  OutputType=Complex  PSBequivalent=0
  Voltage Measurement2 : spsVoltageMeasurementLib/Voltage Measurement  PhasorSimulation=off  OutputType=Complex  PSBequivalent=0
  A : PMIOPort  Side=Left
  B : PMIOPort  Port=2  Side=Left
  C : PMIOPort  Port=3  Side=Left
  wires:
  [Ic] -> I_c/1
  [Ib] -> I_b/1
  PQ/1 -> Calculate Current/1(PQ)
  Demux/3 -> [Ic]
  [Vc] -> Mux/3
  [Vb] -> Mux/2
  Voltage Measurement2/1 -> [Vc]
  [Ia] -> I_a/1
  Calculate Current/1(Iabc) -> Demux/1
  Demux/1 -> [Ia]
  [Va] -> Mux/1
  Voltage Measurement1/1 -> [Vb]
  Mux/1 -> Calculate Current/2(Vabc)  "Vabc"
  Demux/2 -> [Ib]
  Voltage Measurement/1 -> [Va]
  connections:
  Voltage Measurement2/LConn2 -- I_c/RConn1 -- Voltage Measurement1/LConn2 -- I_b/RConn1 -- I_a/RConn1 -- Voltage Measurement/LConn2 -- Ground/LConn1
  C/RConn1 -- I_c/LConn1 -- Voltage Measurement2/LConn1 -- Shunt (Numerical Stability)/LConn3
  B/RConn1 -- Voltage Measurement1/LConn1 -- I_b/LConn1 -- Shunt (Numerical Stability)/LConn2
  A/RConn1 -- I_a/LConn1 -- Voltage Measurement/LConn1 -- Shunt (Numerical Stability)/LConn1
  Ground1/LConn1 -- Shunt (Numerical Stability)/RConn2 -- Shunt (Numerical Stability)/RConn1 -- Shunt (Numerical Stability)/RConn3

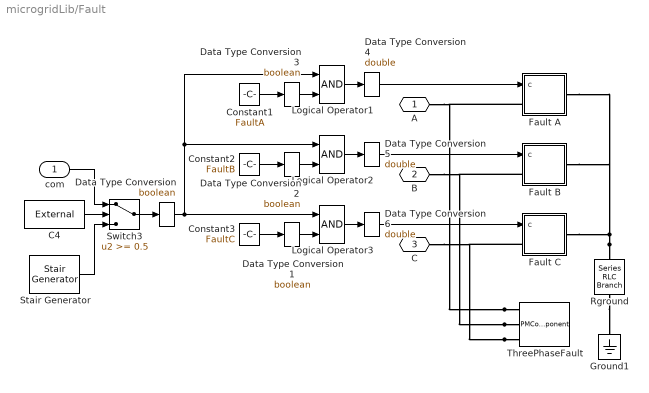
== system microgridLib/Fault  ==
  com : Inport
  C4 : Constant  Value=External
  Constant1 : Constant  Value=FaultA
  Constant2 : Constant  Value=FaultB
  Constant3 : Constant  Value=FaultC
  Data Type Conversion{,1..3} (4 alike) : DataTypeConversion  OutDataTypeStr=boolean
  Data Type Conversion4 : DataTypeConversion  OutDataTypeStr=double
  Data Type Conversion5 : DataTypeConversion  OutDataTypeStr=double
  Data Type Conversion6 : DataTypeConversion  OutDataTypeStr=double
  Fault A : Subsystem  DialogController=POWERSYS.PowerSysDialog  LoadFcn=sps_rtmsupport('LoadFcn',gcbh);  StartFcn=sps_rtmsupport('StartFcn',gcbh);  StopFcn=sps_rtmsupport('StopFcn',gcbh);  mask(Breaker){InitialState=InitialStates(1)*FaultA, SwitchingTimes=[ 1/60  5/60 ], External=on, BreakerResistance=FaultResistance, SnubberResistance=SnubberResistance, SnubberCapacitance=SnubberCapacitance, Measurements=Branch current, MoreParameters=off, NoBreakLoop=off}
      mask prompts: InitialState "Initial status:"; SwitchingTimes "Switching times (s):"; BreakerResistance "Breaker resistance Ron (Ohm):"; SnubberResistance "Snubber resistance Rs (Ohm):"; SnubberCapacitance "Snubber capacitance Cs (F):"; MoreParameters "obsolete"; NoBreakLoop "Enable zero crossing detection (create an algebraic loop)"
      mask help: Implements a circuit breaker. When the external switching time option is selected, a Simulink logical signal is used to control the breaker operation.
      mask init:
      | block = gcb;
      | [WantBlockChoice,Ts,X,Y,BR,Ron] = powericon('SwitchesInit','Breaker',block,SnubberResistance,SnubberCapacitance,BreakerResistance,InitialState,SwitchingTimes,External);
      | %powericon('SetInternalModels','set',block,WantBlockChoice);
      settings: CopyFcn=sps_rtmsupport('CopyFcn',gcbh); powericon('SwitchesCopyFcn','Breaker',gcb)  DeleteFcn=sps_rtmsupport('DeleteFcn',gcbh);  UndoDeleteFcn=sps_rtmsupport('UndoDeleteFcn',gcbh);  ModelCloseFcn=sps_rtmsupport('ModelCloseFcn',gcbh);  PreSaveFcn=sps_rtmsupport('PreSaveFcn',gcbh);  PostSaveFcn=sps_rtmsupport('PostSaveFcn',gcbh);  NameChangeFcn=sps_rtmsupport('NameChangeFcn',gcbh);  PreCopyFcn=sps_rtmsupport('PreCopyFcn',gcbh);  OpenFcn=sps_rtmsupport('OpenFcn',gcbh, [3 7 8 9]);  CloseFcn=sps_rtmsupport('CloseFcn',gcbh);  PreDeleteFcn=sps_rtmsupport('PreDeleteFcn',gcbh);
      mask Help: helpview(psbhelp);
      mask Callback External: powericon('BreakerCback',gcb);
      mask Callback BreakerResistance: powericon('SwitchesEnables',gcb,'Breaker');
      mask TypeOptions Measurements: None | Branch voltage | Branch current | Branch voltage and current
      mask Display: % plot(X.p1,Y.p1,X.p2,Y.p2,X.p3,Y.p3,X.p4,Y.p4,X.p5,Y.p5,X.p6,Y.p6)
  Fault B : Subsystem  DialogController=POWERSYS.PowerSysDialog  LoadFcn=sps_rtmsupport('LoadFcn',gcbh);  StartFcn=sps_rtmsupport('StartFcn',gcbh);  StopFcn=sps_rtmsupport('StopFcn',gcbh);  mask(Breaker){InitialState=InitialStates(1)*FaultB, SwitchingTimes=[ 1/60  5/60 ], External=on, BreakerResistance=FaultResistance, SnubberResistance=SnubberResistance, SnubberCapacitance=SnubberCapacitance, Measurements=Branch current, MoreParameters=off, NoBreakLoop=off}
      mask prompts: InitialState "Initial status:"; SwitchingTimes "Switching times (s):"; BreakerResistance "Breaker resistance Ron (Ohm):"; SnubberResistance "Snubber resistance Rs (Ohm):"; SnubberCapacitance "Snubber capacitance Cs (F):"; MoreParameters "obsolete"; NoBreakLoop "Enable zero crossing detection (create an algebraic loop)"
      mask help: Implements a circuit breaker. When the external switching time option is selected, a Simulink logical signal is used to control the breaker operation.
      mask init: same as microgridLib/Fault /Fault A
      settings: CopyFcn=sps_rtmsupport('CopyFcn',gcbh); powericon('SwitchesCopyFcn','Breaker',gcb)  DeleteFcn=sps_rtmsupport('DeleteFcn',gcbh);  UndoDeleteFcn=sps_rtmsupport('UndoDeleteFcn',gcbh);  ModelCloseFcn=sps_rtmsupport('ModelCloseFcn',gcbh);  PreSaveFcn=sps_rtmsupport('PreSaveFcn',gcbh);  PostSaveFcn=sps_rtmsupport('PostSaveFcn',gcbh);  NameChangeFcn=sps_rtmsupport('NameChangeFcn',gcbh);  PreCopyFcn=sps_rtmsupport('PreCopyFcn',gcbh);  OpenFcn=sps_rtmsupport('OpenFcn',gcbh, [3 7 8 9]);  CloseFcn=sps_rtmsupport('CloseFcn',gcbh);  PreDeleteFcn=sps_rtmsupport('PreDeleteFcn',gcbh);
      mask Help: helpview(psbhelp);
      mask Callback External: powericon('BreakerCback',gcb);
      mask Callback BreakerResistance: powericon('SwitchesEnables',gcb,'Breaker');
      mask TypeOptions Measurements: None | Branch voltage | Branch current | Branch voltage and current
      mask Display: % plot(X.p1,Y.p1,X.p2,Y.p2,X.p3,Y.p3,X.p4,Y.p4,X.p5,Y.p5,X.p6,Y.p6)
  Fault C : Subsystem  DialogController=POWERSYS.PowerSysDialog  LoadFcn=sps_rtmsupport('LoadFcn',gcbh);  StartFcn=sps_rtmsupport('StartFcn',gcbh);  StopFcn=sps_rtmsupport('StopFcn',gcbh);  mask(Breaker){InitialState=InitialStates(1)*FaultC, SwitchingTimes=[ 1/60  5/60 ], External=on, BreakerResistance=FaultResistance, SnubberResistance=SnubberResistance, SnubberCapacitance=SnubberCapacitance, Measurements=Branch current, MoreParameters=off, NoBreakLoop=off}
      mask prompts: InitialState "Initial status:"; SwitchingTimes "Switching times (s):"; BreakerResistance "Breaker resistance Ron (Ohm):"; SnubberResistance "Snubber resistance Rs (Ohm):"; SnubberCapacitance "Snubber capacitance Cs (F):"; MoreParameters "obsolete"; NoBreakLoop "Enable zero crossing detection (create an algebraic loop)"
      mask help: Implements a circuit breaker. When the external switching time option is selected, a Simulink logical signal is used to control the breaker operation.
      mask init: same as microgridLib/Fault /Fault A
      settings: CopyFcn=sps_rtmsupport('CopyFcn',gcbh); powericon('SwitchesCopyFcn','Breaker',gcb)  DeleteFcn=sps_rtmsupport('DeleteFcn',gcbh);  UndoDeleteFcn=sps_rtmsupport('UndoDeleteFcn',gcbh);  ModelCloseFcn=sps_rtmsupport('ModelCloseFcn',gcbh);  PreSaveFcn=sps_rtmsupport('PreSaveFcn',gcbh);  PostSaveFcn=sps_rtmsupport('PostSaveFcn',gcbh);  NameChangeFcn=sps_rtmsupport('NameChangeFcn',gcbh);  PreCopyFcn=sps_rtmsupport('PreCopyFcn',gcbh);  OpenFcn=sps_rtmsupport('OpenFcn',gcbh, [3 7 8 9]);  CloseFcn=sps_rtmsupport('CloseFcn',gcbh);  PreDeleteFcn=sps_rtmsupport('PreDeleteFcn',gcbh);
      mask Help: helpview(psbhelp);
      mask Callback External: powericon('BreakerCback',gcb);
      mask Callback BreakerResistance: powericon('SwitchesEnables',gcb,'Breaker');
      mask TypeOptions Measurements: None | Branch voltage | Branch current | Branch voltage and current
      mask Display: % plot(X.p1,Y.p1,X.p2,Y.p2,X.p3,Y.p3,X.p4,Y.p4,X.p5,Y.p5,X.p6,Y.p6)
  Ground1 : spsGroundLib/Ground  LConnTagsString=a
  Logical Operator1 : Logic
  Logical Operator2 : Logic
  Logical Operator3 : Logic
  Rground : spsSeriesRLCBranchLib/Series RLC Branch  LConnTagsString=__new0  RConnTagsString=__new0  BranchType=R  Resistance=GroundResistance  Inductance=0  SetiL0=off  InitialCurrent=0  Capacitance=inf  Setx0=off  InitialVoltage=0  Measurements=None
  Stair Generator : spsStairGeneratorLib/Stair Generator  t=SwitchTimes  e=SwitchStatus  Ts=Ts
  Switch3 : Switch  Threshold=0.5  ZeroCross=off  SaturateOnIntegerOverflow=off
  ThreePhaseFault : PMComponent  PhysicalDomain=powersysdomain  LeftPortType=p1  RightPortType=p1  LConnTagsString=A|B|C  mask(InnerPowersysBlock){}
  A : PMIOPort  Side=Left
  B : PMIOPort  Port=2  Side=Left
  C : PMIOPort  Port=3  Side=Left
  wires:
  com/1 -> Switch3/1
  Stair Generator/1 -> Switch3/3
  C4/1 -> Switch3/2
  Switch3/1 -> Data Type Conversion/1
  Data Type Conversion/1 -> Logical Operator3/1, Logical Operator2/1, Logical Operator1/1
  Constant3/1 -> Data Type Conversion1/1
  Data Type Conversion1/1 -> Logical Operator3/2
  Constant2/1 -> Data Type Conversion2/1
  Data Type Conversion2/1 -> Logical Operator2/2
  Constant1/1 -> Data Type Conversion3/1
  Data Type Conversion3/1 -> Logical Operator1/2
  Logical Operator1/1 -> Data Type Conversion4/1
  Logical Operator2/1 -> Data Type Conversion5/1
  Logical Operator3/1 -> Data Type Conversion6/1
  Data Type Conversion4/1 -> Fault A/1(c)
  Data Type Conversion5/1 -> Fault B/1(c)
  Data Type Conversion6/1 -> Fault C/1(c)
  connections:
  Rground/RConn1 -- Ground1/LConn1
  ThreePhaseFault/LConn1 -- Fault A/LConn1 -- A/RConn1
  ThreePhaseFault/LConn2 -- Fault B/LConn1 -- B/RConn1
  ThreePhaseFault/LConn3 -- Fault C/LConn1 -- C/RConn1
  Rground/LConn1 -- Fault C/RConn1 -- Fault A/RConn1 -- Fault B/RConn1

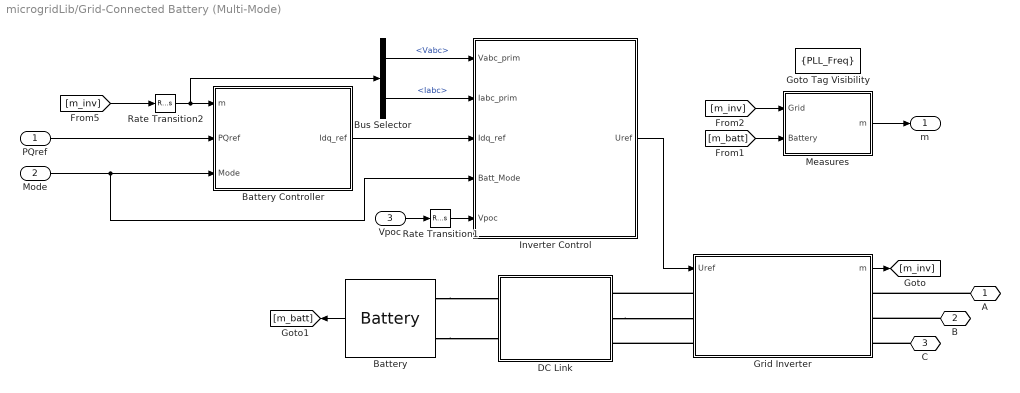
== system microgridLib/Grid-Connected Battery (Multi-Mode) ==
  PQref : Inport  SampleTime=Ts_Control
  Mode : Inport  Port=2
  Vpoc : Inport  Port=3
  Battery : spsBatteryLib/Battery  BatType=Lithium-Ion  ShowTempParam=off  ThermalPreset=no  ShowAgeParam=off  NomV=Vnom_dc  NomQ=Bcap  SOC=75  Batt_Tr=30  PresetModel=on  MaxQ=500  MinV=360  FullV=558.7138  Dis_rate=217.3913  R=0.0096  Normal_OP=452.1739  expZone="[518.5852      24.56522]"  current=[6.5 13 32.5]  Units=Time  Tci=20  NomT=25  T2=0  MaxQ2=2.208  FullV2=3.45  Normal_OP2=2.8  expZone2="[3.22        0.23]"  Rca=0.6  ti=1000  Dp=0  Neq0=0  Tsim=1e6  Ta1=25  Qeol=5.4*0.9  Reol=0.013333*1.2  Char_age=[2.3478, 3]  Dis_age=[2.3478, 10]  N1=1500  N2=10500  N3=1000  N4=1400  Ta2=45  N5=950
      settings: LibrarySourceBlock=electricdrivelib/Extra Sources/Battery
  Battery Controller : Subsystem  SystemSampleTime=Ts
  Bus Selector : BusSelector  OutputSignals=Vabc,Iabc
  DC Link : Subsystem
  Goto Tag Visibility : GotoTagVisibility  GotoTag=PLL_Freq
  Grid Inverter : Subsystem
  Inverter Control : Subsystem
  Measures : Subsystem
  Rate Transition1 : RateTransition  OutPortSampleTime=Ts_Control
  Rate Transition2 : RateTransition  OutPortSampleTime=Ts_Control
  A : PMIOPort  Side=Right
  B : PMIOPort  Port=2  Side=Right
  C : PMIOPort  Port=3  Side=Right
  m : Outport
  wires:
  Rate Transition1/1 -> Inverter Control/5(Vpoc)
  Vpoc/1 -> Rate Transition1/1
  Mode/1 -> Inverter Control/4(Batt_Mode), Battery Controller/3(Mode)
  PQref/1 -> Battery Controller/2(PQref)
  Rate Transition2/1 -> Bus Selector/1, Battery Controller/1(m)
  Inverter Control/1(Uref) -> Grid Inverter/1(Uref)
  Bus Selector/1 -> Inverter Control/1(Vabc_prim)  "<Vabc>"
  Bus Selector/2 -> Inverter Control/2(Iabc_prim)  "<Iabc>"
  Grid Inverter/1(m) -> [m_inv]
  [m_inv] -> Measures/1(Grid)
  [m_batt] -> Measures/2(Battery)
  Measures/1(m) -> m/1
  Battery/1 -> [m_batt]
  [m_inv] -> Rate Transition2/1
  Battery Controller/1(Idq_ref) -> Inverter Control/3(Idq_ref)
  connections:
  Battery/LConn1 -- DC Link/LConn1
  Battery/LConn2 -- DC Link/LConn2
  Grid Inverter/LConn3 -- DC Link/RConn3
  A/RConn1 -- Grid Inverter/RConn1
  B/RConn1 -- Grid Inverter/RConn2
  C/RConn1 -- Grid Inverter/RConn3
  Grid Inverter/LConn1 -- DC Link/RConn1
  DC Link/RConn2 -- Grid Inverter/LConn2

== system microgridLib/Grid-Connected Battery (Simple PQ Only) ==
  PQref : Inport  SampleTime=Ts_Control
  Battery : spsBatteryLib/Battery  BatType=Lithium-Ion  ShowTempParam=off  ThermalPreset=no  ShowAgeParam=off  NomV=Vnom_dc  NomQ=Bcap  SOC=75  Batt_Tr=30  PresetModel=on  MaxQ=500  MinV=360  FullV=558.7138  Dis_rate=217.3913  R=0.0096  Normal_OP=452.1739  expZone="[518.5852      24.56522]"  current=[6.5 13 32.5]  Units=Time  Tci=20  NomT=25  T2=0  MaxQ2=2.208  FullV2=3.45  Normal_OP2=2.8  expZone2="[3.22        0.23]"  Rca=0.6  ti=1000  Dp=0  Neq0=0  Tsim=1e6  Ta1=25  Qeol=5.4*0.9  Reol=0.013333*1.2  Char_age=[2.3478, 3]  Dis_age=[2.3478, 10]  N1=1500  N2=10500  N3=1000  N4=1400  Ta2=45  N5=950
      settings: LibrarySourceBlock=electricdrivelib/Extra Sources/Battery
  Battery Controller : Subsystem  SystemSampleTime=Ts
  Bus Selector : BusSelector  OutputSignals=Vabc,Iabc
  DC Link : Subsystem
  Grid Inverter : Subsystem
  Inverter Control : Subsystem
  Measures : Subsystem
  Rate Transition2 : RateTransition  OutPortSampleTime=Ts_Control
  A : PMIOPort  Side=Right
  B : PMIOPort  Port=2  Side=Right
  C : PMIOPort  Port=3  Side=Right
  m : Outport
  wires:
  PQref/1 -> Battery Controller/2(PQref)
  Rate Transition2/1 -> Battery Controller/1(m), Bus Selector/1
  Inverter Control/1(Uref) -> Grid Inverter/1(Uref)
  Bus Selector/1 -> Inverter Control/1(Vabc_prim)  "<Vabc>"
  Bus Selector/2 -> Inverter Control/2(Iabc_prim)  "<Iabc>"
  Grid Inverter/1(m) -> [m_inv]
  [m_inv] -> Measures/1(Grid)
  [m_batt] -> Measures/2(Battery)
  Measures/1(m) -> m/1
  Battery/1 -> [m_batt]
  [m_inv] -> Rate Transition2/1
  Battery Controller/1(Idq_ref) -> Inverter Control/3(Idq_ref)
  connections:
  Battery/LConn1 -- DC Link/LConn1
  Battery/LConn2 -- DC Link/LConn2
  Grid Inverter/LConn3 -- DC Link/RConn3
  A/RConn1 -- Grid Inverter/RConn1
  B/RConn1 -- Grid Inverter/RConn2
  C/RConn1 -- Grid Inverter/RConn3
  Grid Inverter/LConn1 -- DC Link/RConn1
  DC Link/RConn2 -- Grid Inverter/LConn2

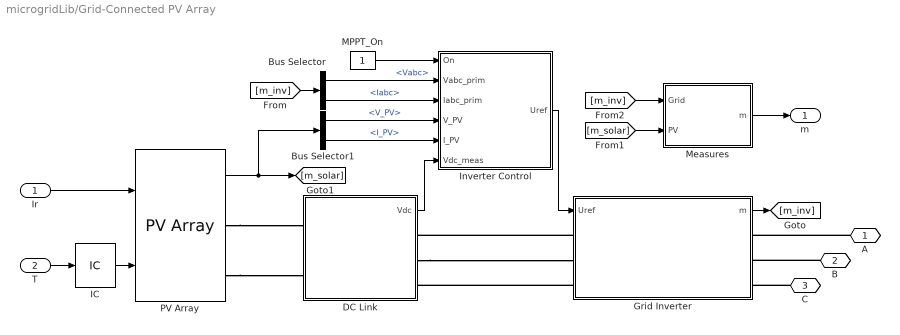
== system microgridLib/Grid-Connected PV Array ==
  Ir : Inport
  T : Inport  Port=2
  Bus Selector : BusSelector  OutputSignals=Vabc,Iabc
  Bus Selector1 : BusSelector  OutputSignals=V_PV,I_PV
  DC Link : Subsystem
  Grid Inverter : Subsystem
  IC : InitialCondition  Value=45
  Inverter Control : Subsystem
  MPPT_On : Constant
  Measures : Subsystem
  PV Array : spsPVArrayLib/PV Array  Npar=round(35*Pmod)  Nser=7  PlotType=array @ 1000 W/m2 & specified temperatures  S_vec="[ 1000  500  100 ]"  Temp_C_vec="[ 45 25  ]"  ModuleName=SunPower SPR-415E-WHT-D  PlotWhenSelected=off  Pm=414.801  Ncell=128  Voc=85.3  Isc=6.09  Vm=72.9  Im=5.69  beta_Voc_pc=-0.229  alpha_Isc_pc=0.030706  beta_Voc=-0.19534  alpha_Isc=0.00187  IL=6.0978  I0=7.1698e-13  nI=0.87223  Rsh=419.7781  Rs=0.53711  RobustModel=off  RobustCellTemperature=313.3991  BAL=on  Tc=1e-6  Tfilter=5e-5
      settings: AttributesFormatString=|
      | %<ModuleName>
      | %<Nser>-module string
      | %<Npar> parallel strings
  A : PMIOPort  Side=Right
  B : PMIOPort  Port=2  Side=Right
  C : PMIOPort  Port=3  Side=Right
  m : Outport
  wires:
  Measures/1(m) -> m/1
  [m_solar] -> Measures/2(PV)
  [m_inv] -> Measures/1(Grid)
  IC/1 -> PV Array/2
  PV Array/1 -> Bus Selector1/1, [m_solar]
  DC Link/1(Vdc) -> Inverter Control/6(Vdc_meas)
  [m_inv] -> Bus Selector/1
  Grid Inverter/1(m) -> [m_inv]
  T/1 -> IC/1
  MPPT_On/1 -> Inverter Control/1(On)
  Bus Selector/2 -> Inverter Control/3(Iabc_prim)  "<Iabc>"
  Bus Selector/1 -> Inverter Control/2(Vabc_prim)  "<Vabc>"
  Bus Selector1/2 -> Inverter Control/5(I_PV)  "<I_PV>"
  Bus Selector1/1 -> Inverter Control/4(V_PV)  "<V_PV>"
  Inverter Control/1(Uref) -> Grid Inverter/1(Uref)
  Ir/1 -> PV Array/1
  connections:
  DC Link/RConn2 -- Grid Inverter/LConn2
  Grid Inverter/LConn1 -- DC Link/RConn1
  C/RConn1 -- Grid Inverter/RConn3
  B/RConn1 -- Grid Inverter/RConn2
  A/RConn1 -- Grid Inverter/RConn1
  Grid Inverter/LConn3 -- DC Link/RConn3
  PV Array/RConn2 -- DC Link/LConn2
  PV Array/RConn1 -- DC Link/LConn1

== system microgridLib/Line  ==
  A : PMIOPort  Side=Left
  a : PMIOPort  Port=2  Side=Right
  B : PMIOPort  Port=3  Side=Left
  b : PMIOPort  Port=4  Side=Right
  C : PMIOPort  Port=5  Side=Left
  c : PMIOPort  Port=6  Side=Right
  connections:
  A/RConn1 -- a/RConn1
  B/RConn1 -- b/RConn1
  C/RConn1 -- c/RConn1

== system microgridLib/Line (Series) ==
  Series Impedance : spsThreePhaseSeriesRLCBranchLib/Three-Phase Series RLC Branch  LConnTagsString=A|B|C  RConnTagsString=A|B|C  BranchType=RL  Resistance=R0*Length  Inductance=L0*Length  Capacitance=0  Measurements=None
  A : PMIOPort  Side=Left
  a : PMIOPort  Port=2  Side=Right
  B : PMIOPort  Port=3  Side=Left
  b : PMIOPort  Port=4  Side=Right
  C : PMIOPort  Port=5  Side=Left
  c : PMIOPort  Port=6  Side=Right
  connections:
  A/RConn1 -- Series Impedance/RConn1
  B/RConn1 -- Series Impedance/RConn2
  C/RConn1 -- Series Impedance/RConn3
  Series Impedance/LConn1 -- a/RConn1
  Series Impedance/LConn2 -- b/RConn1
  Series Impedance/LConn3 -- c/RConn1

== system microgridLib/Relay ==
  Input : Inport
  " Shunt (Numerical Stability)" : spsThreePhaseSeriesRLCBranchLib/Three-Phase Series RLC Branch  LConnTagsString=A|B|C  RConnTagsString=A|B|C  BranchType=R  Resistance=1e7  Inductance=1e-3  Capacitance=1e-6  Measurements=None
  Breaker (Pure Discrete) : Subsystem  Commented=on  DialogController=POWERSYS.PowerSysDialog  LoadFcn=sps_rtmsupport('LoadFcn',gcbh);  StartFcn=sps_rtmsupport('StartFcn',gcbh);  StopFcn=sps_rtmsupport('StopFcn',gcbh);  mask(Three-Phase Breaker){InitialState=closed, SwitchA=on, SwitchB=on, SwitchC=on, SwitchTimes=2/60, External=on, BreakerResistance=1e-4, SnubberResistance=1e15, SnubberCapacitance=inf, Measurements=None}
      mask prompts: InitialState "Initial status:"; SwitchA "Phase A"; SwitchB "Phase B"; SwitchC "Phase C"; SwitchTimes "Switching times (s):"; BreakerResistance "Breaker resistance Ron (Ohm):"; SnubberResistance "Snubber resistance Rs (Ohm):"; SnubberCapacitance "Snubber capacitance Cs (F):"
      mask help: Implements a three-phase circuit breaker. When the external switching time mode is selected, a Simulink logical signal is used to control the breaker operation.
      mask init:
      | block = gcb;
      | [X,Y,SwitchStatus,InitialState,Ts,Switch_Times] = powericon('ThreePhaseBreakerInit',block,InitialState,SwitchTimes,External,SnubberResistance,SnubberCapacitance);
      | powericon('ThreePhaseBreakerCback',block);
      settings: CopyFcn=sps_rtmsupport('CopyFcn',gcbh);  DeleteFcn=sps_rtmsupport('DeleteFcn',gcbh);  UndoDeleteFcn=sps_rtmsupport('UndoDeleteFcn',gcbh);  ModelCloseFcn=sps_rtmsupport('ModelCloseFcn',gcbh);  PreSaveFcn=sps_rtmsupport('PreSaveFcn',gcbh);  PostSaveFcn=sps_rtmsupport('PostSaveFcn',gcbh);  NameChangeFcn=sps_rtmsupport('NameChangeFcn',gcbh);  PreCopyFcn=sps_rtmsupport('PreCopyFcn',gcbh);  OpenFcn=sps_rtmsupport('OpenFcn',gcbh, [1 2 3 4 6 10]);  CloseFcn=sps_rtmsupport('CloseFcn',gcbh);  PreDeleteFcn=sps_rtmsupport('PreDeleteFcn',gcbh);
      mask Help: helpview(psbhelp)
      mask TypeOptions InitialState: open | closed
      mask Callback External: powericon('ThreePhaseBreakerCback',gcb);
      mask TypeOptions Measurements: None | Breaker voltages | Breaker currents | Breaker voltages and currents
      mask DialogControl Container3 Prompt: Switching of:
      mask Display: plot(X.p1,Y.p1,X.p2,Y.p2,X.p3,Y.p3,X.p4,Y.p4,X.p5,Y.p5,X.p6,Y.p6)
  Breaker (SPS Default) : spsThreePhaseBreakerLib/Three-Phase Breaker  InitialState=closed  SwitchA=on  SwitchB=on  SwitchC=on  SwitchTimes="[1/60  5/60]"  External=on  BreakerResistance=1e-4  SnubberResistance=1e15  SnubberCapacitance=inf  Measurements=None
  Ground : spsGroundLib/Ground  LConnTagsString=a
  Ground1 : spsGroundLib/Ground  LConnTagsString=a
  Ground2 : Ground
  Shunt (Numerical Stability) : spsThreePhaseSeriesRLCBranchLib/Three-Phase Series RLC Branch  LConnTagsString=A|B|C  RConnTagsString=A|B|C  BranchType=R  Resistance=1e7  Inductance=1e-3  Capacitance=1e-6  Measurements=None
  A : PMIOPort  Tag=PMCPort  Side=Left
  B : PMIOPort  Tag=PMCPort  Port=2  Side=Left
  C : PMIOPort  Tag=PMCPort  Port=3  Side=Left
  a : PMIOPort  Tag=PMCPort  Port=4  Side=Right
  b : PMIOPort  Tag=PMCPort  Port=5  Side=Right
  c : PMIOPort  Tag=PMCPort  Port=6  Side=Right
  m : Outport
  wires:
  Input/1 -> Breaker (SPS Default)/1
  Ground2/1 -> m/1
  connections:
  Shunt (Numerical Stability)/RConn3 -- Ground/LConn1 -- Shunt (Numerical Stability)/RConn2 -- Shunt (Numerical Stability)/RConn1
  Shunt (Numerical Stability)/LConn1 -- Breaker (SPS Default)/LConn1 -- A/RConn1
  Shunt (Numerical Stability)/LConn2 -- Breaker (SPS Default)/LConn2 -- B/RConn1
  " Shunt (Numerical Stability)"/LConn3 -- Breaker (SPS Default)/RConn3 -- c/RConn1
  " Shunt (Numerical Stability)"/RConn3 -- Ground1/LConn1 -- " Shunt (Numerical Stability)"/RConn1 -- " Shunt (Numerical Stability)"/RConn2
  " Shunt (Numerical Stability)"/LConn2 -- Breaker (SPS Default)/RConn2 -- b/RConn1
  " Shunt (Numerical Stability)"/LConn1 -- Breaker (SPS Default)/RConn1 -- a/RConn1
  Shunt (Numerical Stability)/LConn3 -- Breaker (SPS Default)/LConn3 -- C/RConn1

== system microgridLib/Static Load ==
  Constant Load : spsThreePhaseSeriesRLCLoadLib/Three-Phase Series RLC Load  LConnTagsString=A|B|C  Configuration=Y (grounded)  NominalVoltage=Vrms  Vabc=[1e3 1e3 1e3]  Vabcp=[1e3 1e3 1e3]  NominalFrequency=Freq  UnbalancedPower=off  ActivePower=S*PF  InductivePower=S*sqrt(1-PF^2)  CapacitivePower=0  Pabc=[10e3 9e3 11e3]  QLabc=[100 90 110]  QCabc=[100 90 110]  Pabcp=[10e3 9e3 11e3]  QLabcp=[100 90 110]  QCabcp=[100 90 110]  Measurements=None  LoadType=constant Z
  A : PMIOPort  Side=Left
  B : PMIOPort  Port=2  Side=Left
  C : PMIOPort  Port=3  Side=Left
  connections:
  Constant Load/LConn3 -- C/RConn1
  Constant Load/LConn1 -- A/RConn1
  Constant Load/LConn2 -- B/RConn1
